simulink library "OPLEV_MASTER"  (Simulink 8.6)
settings: Solver=ode45  StartTime=0.0  StopTime=10.0  RelTol=1e-3
libraries: cdsEpicsOut x9, cdsRms x6, cdsEpicsIn x6
settings Model: Creator=controls  LastModifiedBy=controls

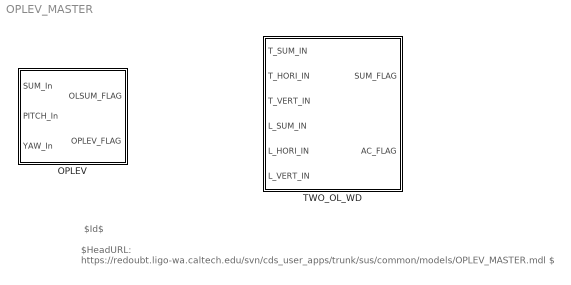
== system OPLEV_MASTER ==
  note: $HeadURL: https://redoubt.ligo-wa.caltech.edu/svn/cds_user_apps/trunk/sus/common/models/OPLEV_MASTER.mdl $
  note: $Id$
  OPLEV : Subsystem
  TWO_OL_WD : Subsystem

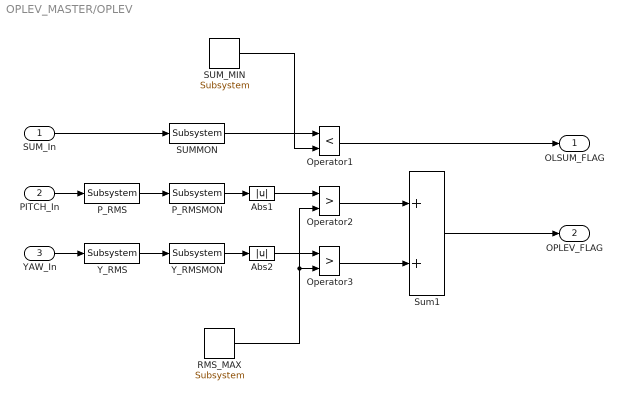
== system OPLEV_MASTER/OPLEV ==
  SUM_In : Inport
  PITCH_In : Inport  Port=2
  YAW_In : Inport  Port=3
  Abs1 : Abs
  Abs2 : Abs
  Operator1 : RelationalOperator  Operator=<  OutDataTypeStr=boolean
  Operator2 : RelationalOperator  Operator=>  OutDataTypeStr=boolean  ZeroCross=off
  Operator3 : RelationalOperator  Operator=>  OutDataTypeStr=boolean
  P_RMS : cdsRms/Subsystem  Tag=cdsRms  Description=|
      | Purpose:
      | Calculate an RMS based on the input signal.
      settings: AttributesFormatString=%<Tag>
  P_RMSMON : cdsEpicsOut/Subsystem  Tag=cdsEpicsOutput  Description=|
      | Purpose:                                          
      | Output a FE signal to an EPICS channel.           
      |                                                   
      | Operation:                                        
      | Takes input value and passes it to EPICS record.  
      |                                                   
      | Usage:                                            
      | Name the part with the desired EPICS rrecord name.
      settings: AttributesFormatString=%<Tag>
  RMS_MAX : cdsEpicsIn/Subsystem  Tag=cdsEpicsIn  Description=|
      | Purpose:                                                                              
      | Create an EPICS input channel connection to the FE realtime controls.                 
      |                                                                                       
      | Operation:                                                                            
      | Outputs value from an EPICS ai record. Value is floating point with a precision of 3..
      |                                                                                       
      | Usage:                                                                                
      | Name the part with the desired EPICS channel name.
      settings: AttributesFormatString=%<Tag>
  SUMMON : cdsEpicsOut/Subsystem  Tag=cdsEpicsOutput  Description=|
      | Purpose:                                          
      | Output a FE signal to an EPICS channel.           
      |                                                   
      | Operation:                                        
      | Takes input value and passes it to EPICS record.  
      |                                                   
      | Usage:                                            
      | Name the part with the desired EPICS rrecord name.
      settings: AttributesFormatString=%<Tag>
  SUM_MIN : cdsEpicsIn/Subsystem  Tag=cdsEpicsIn  Description=|
      | Purpose:                                                                              
      | Create an EPICS input channel connection to the FE realtime controls.                 
      |                                                                                       
      | Operation:                                                                            
      | Outputs value from an EPICS ai record. Value is floating point with a precision of 3..
      |                                                                                       
      | Usage:                                                                                
      | Name the part with the desired EPICS channel name.
      settings: AttributesFormatString=%<Tag>
  Sum1 : Sum
  Y_RMS : cdsRms/Subsystem  Tag=cdsRms  Description=|
      | Purpose:
      | Calculate an RMS based on the input signal.
      settings: AttributesFormatString=%<Tag>
  Y_RMSMON : cdsEpicsOut/Subsystem  Tag=cdsEpicsOutput  Description=|
      | Purpose:                                          
      | Output a FE signal to an EPICS channel.           
      |                                                   
      | Operation:                                        
      | Takes input value and passes it to EPICS record.  
      |                                                   
      | Usage:                                            
      | Name the part with the desired EPICS rrecord name.
      settings: AttributesFormatString=%<Tag>
  OLSUM_FLAG : Outport
  OPLEV_FLAG : Outport  Port=2
  wires:
  Operator1/1 -> OLSUM_FLAG/1
  Operator3/1 -> Sum1/2
  Operator2/1 -> Sum1/1
  Y_RMSMON/1 -> Abs2/1
  P_RMSMON/1 -> Abs1/1
  SUMMON/1 -> Operator1/1
  Y_RMS/1 -> Y_RMSMON/1
  P_RMS/1 -> P_RMSMON/1
  RMS_MAX/1 -> Operator3/2, Operator2/2
  Sum1/1 -> OPLEV_FLAG/1
  SUM_MIN/1 -> Operator1/2
  YAW_In/1 -> Y_RMS/1
  PITCH_In/1 -> P_RMS/1
  SUM_In/1 -> SUMMON/1
  Abs2/1 -> Operator3/1
  Abs1/1 -> Operator2/1

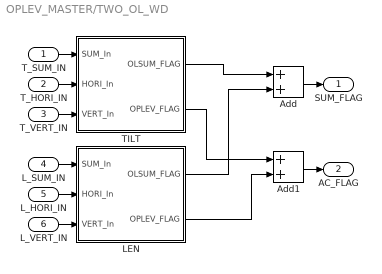
== system OPLEV_MASTER/TWO_OL_WD ==
  T_SUM_IN : Inport
  T_HORI_IN : Inport  Port=2
  T_VERT_IN : Inport  Port=3
  L_SUM_IN : Inport  Port=4
  L_HORI_IN : Inport  Port=5
  L_VERT_IN : Inport  Port=6
  Add : Sum
  Add1 : Sum
  LEN : Subsystem
  TILT : Subsystem
  SUM_FLAG : Outport
  AC_FLAG : Outport  Port=2
  wires:
  LEN/2(OPLEV_FLAG) -> Add1/2
  T_HORI_IN/1 -> TILT/2(HORI_In)
  T_VERT_IN/1 -> TILT/3(VERT_In)
  L_SUM_IN/1 -> LEN/1(SUM_In)
  TILT/1(OLSUM_FLAG) -> Add/1
  Add/1 -> SUM_FLAG/1
  TILT/2(OPLEV_FLAG) -> Add1/1
  L_VERT_IN/1 -> LEN/3(VERT_In)
  T_SUM_IN/1 -> TILT/1(SUM_In)
  Add1/1 -> AC_FLAG/1
  LEN/1(OLSUM_FLAG) -> Add/2
  L_HORI_IN/1 -> LEN/2(HORI_In)

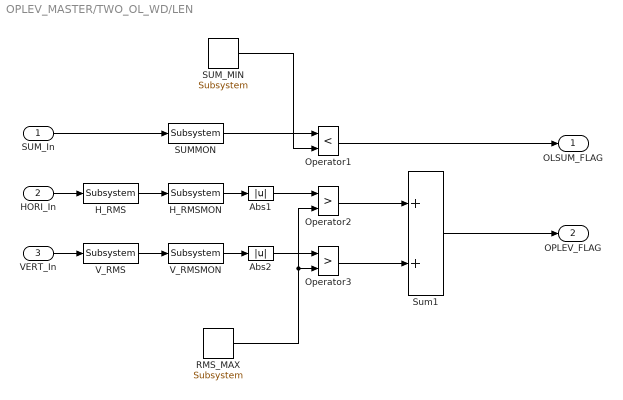
== system OPLEV_MASTER/TWO_OL_WD/LEN ==
  SUM_In : Inport
  HORI_In : Inport  Port=2
  VERT_In : Inport  Port=3
  Abs1 : Abs
  Abs2 : Abs
  H_RMS : cdsRms/Subsystem  Tag=cdsRms  Description=|
      | Purpose:
      | Calculate an RMS based on the input signal.
      settings: AttributesFormatString=%<Tag>
  H_RMSMON : cdsEpicsOut/Subsystem  Tag=cdsEpicsOutput  Description=|
      | Purpose:                                          
      | Output a FE signal to an EPICS channel.           
      |                                                   
      | Operation:                                        
      | Takes input value and passes it to EPICS record.  
      |                                                   
      | Usage:                                            
      | Name the part with the desired EPICS rrecord name.
      settings: AttributesFormatString=%<Tag>
  Operator1 : RelationalOperator  Operator=<  OutDataTypeStr=boolean
  Operator2 : RelationalOperator  Operator=>  OutDataTypeStr=boolean  ZeroCross=off
  Operator3 : RelationalOperator  Operator=>  OutDataTypeStr=boolean
  RMS_MAX : cdsEpicsIn/Subsystem  Tag=cdsEpicsIn  Description=|
      | Purpose:                                                                              
      | Create an EPICS input channel connection to the FE realtime controls.                 
      |                                                                                       
      | Operation:                                                                            
      | Outputs value from an EPICS ai record. Value is floating point with a precision of 3..
      |                                                                                       
      | Usage:                                                                                
      | Name the part with the desired EPICS channel name.
      settings: AttributesFormatString=%<Tag>
  SUMMON : cdsEpicsOut/Subsystem  Tag=cdsEpicsOutput  Description=|
      | Purpose:                                          
      | Output a FE signal to an EPICS channel.           
      |                                                   
      | Operation:                                        
      | Takes input value and passes it to EPICS record.  
      |                                                   
      | Usage:                                            
      | Name the part with the desired EPICS rrecord name.
      settings: AttributesFormatString=%<Tag>
  SUM_MIN : cdsEpicsIn/Subsystem  Tag=cdsEpicsIn  Description=|
      | Purpose:                                                                              
      | Create an EPICS input channel connection to the FE realtime controls.                 
      |                                                                                       
      | Operation:                                                                            
      | Outputs value from an EPICS ai record. Value is floating point with a precision of 3..
      |                                                                                       
      | Usage:                                                                                
      | Name the part with the desired EPICS channel name.
      settings: AttributesFormatString=%<Tag>
  Sum1 : Sum
  V_RMS : cdsRms/Subsystem  Tag=cdsRms  Description=|
      | Purpose:
      | Calculate an RMS based on the input signal.
      settings: AttributesFormatString=%<Tag>
  V_RMSMON : cdsEpicsOut/Subsystem  Tag=cdsEpicsOutput  Description=|
      | Purpose:                                          
      | Output a FE signal to an EPICS channel.           
      |                                                   
      | Operation:                                        
      | Takes input value and passes it to EPICS record.  
      |                                                   
      | Usage:                                            
      | Name the part with the desired EPICS rrecord name.
      settings: AttributesFormatString=%<Tag>
  OLSUM_FLAG : Outport
  OPLEV_FLAG : Outport  Port=2
  wires:
  Operator1/1 -> OLSUM_FLAG/1
  Operator3/1 -> Sum1/2
  Operator2/1 -> Sum1/1
  V_RMSMON/1 -> Abs2/1
  H_RMSMON/1 -> Abs1/1
  SUMMON/1 -> Operator1/1
  V_RMS/1 -> V_RMSMON/1
  H_RMS/1 -> H_RMSMON/1
  RMS_MAX/1 -> Operator3/2, Operator2/2
  Sum1/1 -> OPLEV_FLAG/1
  SUM_MIN/1 -> Operator1/2
  VERT_In/1 -> V_RMS/1
  HORI_In/1 -> H_RMS/1
  SUM_In/1 -> SUMMON/1
  Abs2/1 -> Operator3/1
  Abs1/1 -> Operator2/1

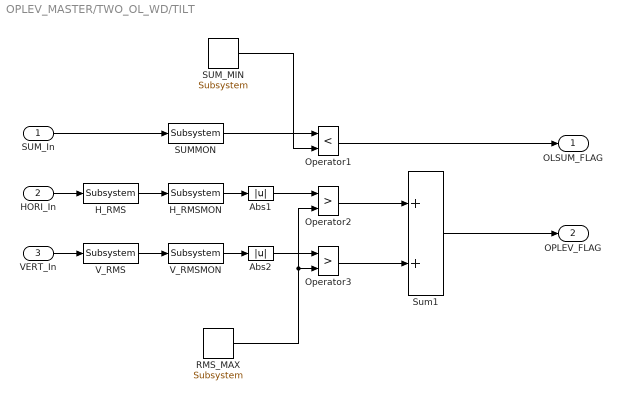
== system OPLEV_MASTER/TWO_OL_WD/TILT ==
  SUM_In : Inport
  HORI_In : Inport  Port=2
  VERT_In : Inport  Port=3
  Abs1 : Abs
  Abs2 : Abs
  H_RMS : cdsRms/Subsystem  Tag=cdsRms  Description=|
      | Purpose:
      | Calculate an RMS based on the input signal.
      settings: AttributesFormatString=%<Tag>
  H_RMSMON : cdsEpicsOut/Subsystem  Tag=cdsEpicsOutput  Description=|
      | Purpose:                                          
      | Output a FE signal to an EPICS channel.           
      |                                                   
      | Operation:                                        
      | Takes input value and passes it to EPICS record.  
      |                                                   
      | Usage:                                            
      | Name the part with the desired EPICS rrecord name.
      settings: AttributesFormatString=%<Tag>
  Operator1 : RelationalOperator  Operator=<  OutDataTypeStr=boolean
  Operator2 : RelationalOperator  Operator=>  OutDataTypeStr=boolean  ZeroCross=off
  Operator3 : RelationalOperator  Operator=>  OutDataTypeStr=boolean
  RMS_MAX : cdsEpicsIn/Subsystem  Tag=cdsEpicsIn  Description=|
      | Purpose:                                                                              
      | Create an EPICS input channel connection to the FE realtime controls.                 
      |                                                                                       
      | Operation:                                                                            
      | Outputs value from an EPICS ai record. Value is floating point with a precision of 3..
      |                                                                                       
      | Usage:                                                                                
      | Name the part with the desired EPICS channel name.
      settings: AttributesFormatString=%<Tag>
  SUMMON : cdsEpicsOut/Subsystem  Tag=cdsEpicsOutput  Description=|
      | Purpose:                                          
      | Output a FE signal to an EPICS channel.           
      |                                                   
      | Operation:                                        
      | Takes input value and passes it to EPICS record.  
      |                                                   
      | Usage:                                            
      | Name the part with the desired EPICS rrecord name.
      settings: AttributesFormatString=%<Tag>
  SUM_MIN : cdsEpicsIn/Subsystem  Tag=cdsEpicsIn  Description=|
      | Purpose:                                                                              
      | Create an EPICS input channel connection to the FE realtime controls.                 
      |                                                                                       
      | Operation:                                                                            
      | Outputs value from an EPICS ai record. Value is floating point with a precision of 3..
      |                                                                                       
      | Usage:                                                                                
      | Name the part with the desired EPICS channel name.
      settings: AttributesFormatString=%<Tag>
  Sum1 : Sum
  V_RMS : cdsRms/Subsystem  Tag=cdsRms  Description=|
      | Purpose:
      | Calculate an RMS based on the input signal.
      settings: AttributesFormatString=%<Tag>
  V_RMSMON : cdsEpicsOut/Subsystem  Tag=cdsEpicsOutput  Description=|
      | Purpose:                                          
      | Output a FE signal to an EPICS channel.           
      |                                                   
      | Operation:                                        
      | Takes input value and passes it to EPICS record.  
      |                                                   
      | Usage:                                            
      | Name the part with the desired EPICS rrecord name.
      settings: AttributesFormatString=%<Tag>
  OLSUM_FLAG : Outport
  OPLEV_FLAG : Outport  Port=2
  wires:
  Operator1/1 -> OLSUM_FLAG/1
  Operator3/1 -> Sum1/2
  Operator2/1 -> Sum1/1
  V_RMSMON/1 -> Abs2/1
  H_RMSMON/1 -> Abs1/1
  SUMMON/1 -> Operator1/1
  V_RMS/1 -> V_RMSMON/1
  H_RMS/1 -> H_RMSMON/1
  RMS_MAX/1 -> Operator3/2, Operator2/2
  Sum1/1 -> OPLEV_FLAG/1
  SUM_MIN/1 -> Operator1/2
  VERT_In/1 -> V_RMS/1
  HORI_In/1 -> H_RMS/1
  SUM_In/1 -> SUMMON/1
  Abs2/1 -> Operator3/1
  Abs1/1 -> Operator2/1
